simulink model "Lib"  (R2015b)
settings: Solver=VariableStepAuto  SolverMode=SingleTasking  StartTime=0.0  StopTime=10.0  RelTol=1e-3
libraries: simulink x2
settings Model: Creator=Castiel  LastModifiedBy=Castiel
settings DataIOCC: LimitDataPoints=off  ReturnWorkspaceOutputs=on
settings DebuggingCC: UnconnectedInputMsg=none  UnconnectedOutputMsg=none  UnconnectedLineMsg=none  AllowSymbolicDim=on  SFUnexpectedBacktrackingDiag=error  SFNoUnconditionalDefaultTransitionDiag=error
settings ModelReferenceCC: PropagateSignalLabelsOutOfModel=on
settings SFSimCC: SimUseLocalCustomCode=on
settings RTWCC: RTWUseLocalCustomCode=on
settings GRTTargetCC: TargetLangStandard=C99 (ISO)
settings ConfigComp: CovMetricSettings=dwe  CovSaveCumulativeToWorkspaceVar=off  CovSaveSingleToWorkspaceVar=off  CovModelRefEnable=Off  CovExternalEMLEnable=on

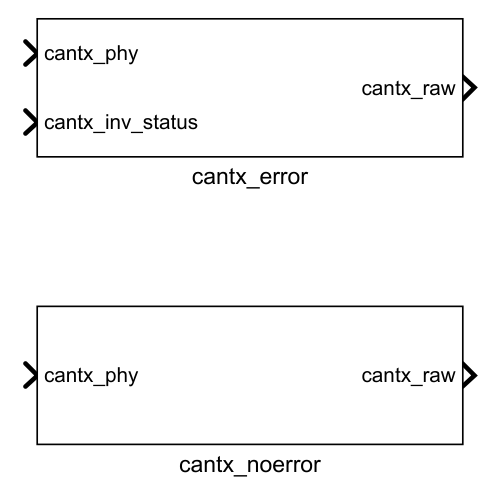
[thumbnail: Simulink's stored preview of the top-level diagram]
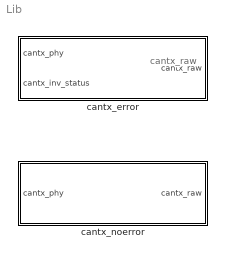
== system Lib ==
  note: cantx_raw
  cantx_error : Subsystem
  cantx_noerror : Subsystem

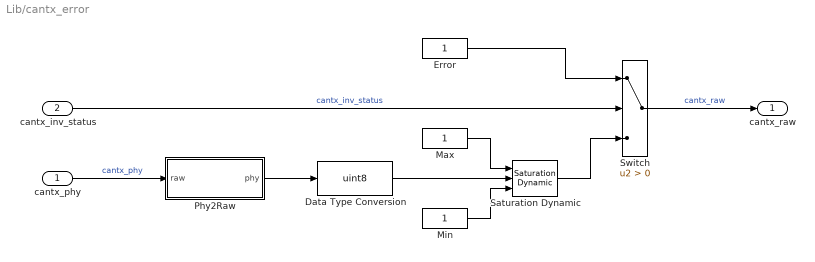
== system Lib/cantx_error ==
  cantx_phy : Inport
  cantx_inv_status : Inport  Port=2
  Data Type Conversion : DataTypeConversion  OutDataTypeStr=uint8
  Error : Constant
  Max : Constant
  Min : Constant
  Phy2Raw : Subsystem  mask{Offset=0, Factor=0}
      mask Callback Offset:
      | offset = get_param(gcb, 'Offset');
      |     set_param([gcb, '/Offset'], 'Value', offset);
      mask Callback Factor:
      | factor = get_param(gcb, 'Factor');
      |     set_param([gcb, '/Factor'], 'Value', factor);
      mask Display:
      | disp(['Offset = ', get_param(gcb, 'Offset'), '\n\n']);
      | disp(['Factor = ', get_param(gcb, 'Factor')]);
  Saturation Dynamic : simulink/Discontinuities/Saturation Dynamic  OutMin=[]  OutMax=[]  OutDataTypeStr=Inherit: Same as second input  OutDataType=fixdt(1, 16)  OutScaling=2^-10  DoSatur=off
  Switch : Switch  Criteria=u2 > Threshold
  cantx_raw : Outport
  wires:
  cantx_inv_status/1 -> Switch/2  "cantx_inv_status"
  Max/1 -> Saturation Dynamic/1
  Error/1 -> Switch/1
  Min/1 -> Saturation Dynamic/3
  cantx_phy/1 -> Phy2Raw/1(raw)  "cantx_phy"
  Data Type Conversion/1 -> Saturation Dynamic/2
  Phy2Raw/1(phy) -> Data Type Conversion/1
  Saturation Dynamic/1 -> Switch/3
  Switch/1 -> cantx_raw/1  "cantx_raw"

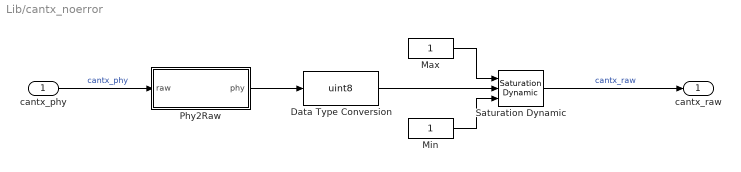
== system Lib/cantx_noerror ==
  cantx_phy : Inport
  Data Type Conversion : DataTypeConversion  OutDataTypeStr=uint8
  Max : Constant
  Min : Constant
  Phy2Raw : Subsystem  mask{Offset=0, Factor=0}
      mask Callback Offset:
      | offset = get_param(gcb, 'Offset');
      |     set_param([gcb, '/Offset'], 'Value', offset);
      mask Callback Factor:
      | factor = get_param(gcb, 'Factor');
      |     set_param([gcb, '/Factor'], 'Value', factor);
      mask Display:
      | disp(['Offset = ', get_param(gcb, 'Offset'), '\n\n']);
      | disp(['Factor = ', get_param(gcb, 'Factor')]);
  Saturation Dynamic : simulink/Discontinuities/Saturation Dynamic  OutMin=[]  OutMax=[]  OutDataTypeStr=Inherit: Same as second input  OutDataType=fixdt(1, 16)  OutScaling=2^-10  DoSatur=off
  cantx_raw : Outport
  wires:
  Max/1 -> Saturation Dynamic/1
  Min/1 -> Saturation Dynamic/3
  cantx_phy/1 -> Phy2Raw/1(raw)  "cantx_phy"
  Data Type Conversion/1 -> Saturation Dynamic/2
  Phy2Raw/1(phy) -> Data Type Conversion/1
  Saturation Dynamic/1 -> cantx_raw/1  "cantx_raw"

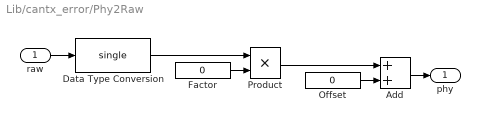
== system Lib/cantx_error/Phy2Raw ==
  raw : Inport
  Add : Sum
  Data Type Conversion : DataTypeConversion  OutDataTypeStr=single
  Factor : Constant  Value=0
  Offset : Constant  Value=0
  Product : Product
  phy : Outport
  wires:
  raw/1 -> Data Type Conversion/1
  Product/1 -> Add/1
  Offset/1 -> Add/2
  Data Type Conversion/1 -> Product/1
  Factor/1 -> Product/2
  Add/1 -> phy/1

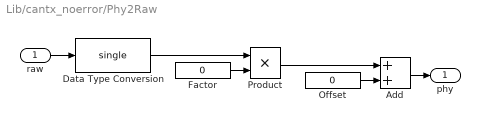
== system Lib/cantx_noerror/Phy2Raw ==
  raw : Inport
  Add : Sum
  Data Type Conversion : DataTypeConversion  OutDataTypeStr=single
  Factor : Constant  Value=0
  Offset : Constant  Value=0
  Product : Product
  phy : Outport
  wires:
  raw/1 -> Data Type Conversion/1
  Product/1 -> Add/1
  Offset/1 -> Add/2
  Data Type Conversion/1 -> Product/1
  Factor/1 -> Product/2
  Add/1 -> phy/1
